simulink model "SimulArm_Interpolate_V2"  (R2025b)
settings: Solver=VariableStepAuto  StartTime=0.0  StopTime=45  FixedStep=.02  RelTol=1e-3  AbsTol=1e-3  EnableMultiTasking=on
values from neighbouring files (symbols this model uses):
  C = U * V'    [DataCondition.m]
  g = 9.80665    [DataCondition.m]
  N = numel(raw)    [DataCondition.m]
  pitch_offset = 0    [DataCondition.m]
  rot_x_bicep = [rot_x_bicep_ramp; rot_x_bicep]    [DataCondition.m]
  rot_y_bicep = [zeros(n_ramp,1); rot_y_bicep]    [DataCondition.m]
  rot_y_wrist = [zeros(n_ramp,1); rot_y_wrist]    [DataCondition.m]
  rot_z_bicep = [zeros(n_ramp,1); rot_z_bicep]    [DataCondition.m]
  rot_z_wrist = [zeros(n_ramp,1); rot_z_wrist]    [DataCondition.m]
  shoulder_limit = 30    [DataCondition.m]
  time = [time_ramp; time_motion]    [DataCondition.m]
  yaw_offset = 0    [DataCondition.m]
undefined symbols (not defined in the file or in its folder): X, Y, Z
libraries: sm_lib x45, nesl_utility x24, aerolibconvert2 x10, simulink x1
(part 3 of 3)

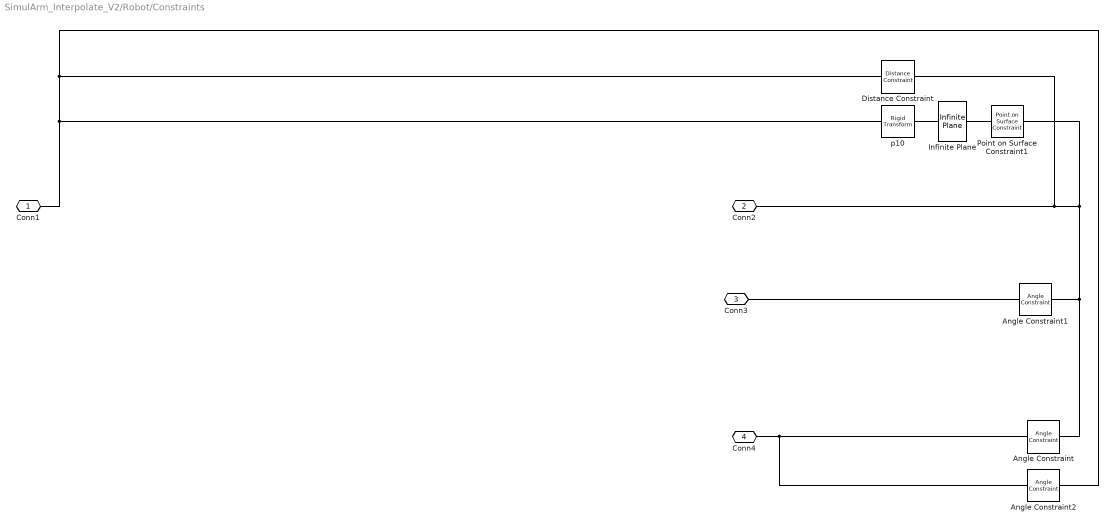
== system SimulArm_Interpolate_V2/Robot/Constraints ==
  Angle Constraint : sm_lib/Constraints/Angle Constraint  ConstraintType=Parallel  Angle=45  AngleUnits=deg  WrenchDir=FollowerOnBase  WrenchFrame=BaseFrame  SenseTorque=off  SenseSignedTorqueMagnitude=off
  Angle Constraint1 : sm_lib/Constraints/Angle Constraint  ConstraintType=Parallel  Angle=45  AngleUnits=deg  WrenchDir=FollowerOnBase  WrenchFrame=BaseFrame  SenseTorque=off  SenseSignedTorqueMagnitude=off
  Angle Constraint2 : sm_lib/Constraints/Angle Constraint  ConstraintType=Parallel  Angle=45  AngleUnits=deg  WrenchDir=FollowerOnBase  WrenchFrame=BaseFrame  SenseTorque=off  SenseSignedTorqueMagnitude=off
  Distance Constraint : sm_lib/Constraints/Distance Constraint  Distance=132  DistanceUnits=mm  WrenchDir=FollowerOnBase  WrenchFrame=BaseFrame  SenseForce=off  SenseSignedForceMagnitude=off
  Infinite Plane : sm_lib/Curves and Surfaces/Infinite Plane  GraphicType=Rectangle  GraphicPlaneWidth=1  GraphicPlaneWidthUnits=m  GraphicPlaneHeight=1  GraphicPlaneHeightUnits=m  GraphicVisPropType=SimpleVisualProperties  GraphicDiffuseColor=[0.5 0.5 0.5]  GraphicOpacity=.3  GraphicSpecularColor=[0.5 0.5 0.5 1.0]  GraphicAmbientColor=[0.15 0.15 0.15 1.0]  GraphicEmissiveColor=[0.0 0.0 0.0 1.0]  GraphicShininess=75
  Point on Surface Constraint1 : sm_lib/Constraints/Point on Surface Constraint  WrenchDir=FollowerOnBase  WrenchFrame=BaseFrame  SenseForce=off  SenseTorque=off
  p10 : sm_lib/Frames and Transforms/Rigid Transform  RotationMethod=None  FollAlignAxisA=+X  BaseAlignAxisA=+Y  FollAlignAxisB=+Y  BaseAlignAxisB=+Z  RotationStandardAxis=+Z  RotationAngle=0.0  RotationAngleUnits=deg  RotationArbitraryAxis=[0 0 1]  RotationSequenceAxes=FollowerAxes  RotationSequence=XZY  RotationSequenceAngles=-[90 -45 0]  RotationSequenceAnglesUnits=deg  RotationMatrix=[1 0 0; 0 1 0; 0 0 1]  Quaternion=[1 0 0 0]  TranslationMethod=Cartesian  TranslationCartesianOffset=[0 0 -132]  TranslationCartesianOffsetUnits=mm  TranslationStandardAxis=+Z  TranslationStandardOffset=0  TranslationStandardOffsetUnits=m  TranslationROffset=0  TranslationROffsetUnits=m  TranslationThetaOffset=0  TranslationThetaOffsetUnits=deg  TranslationZOffset=0  TranslationZOffsetUnits=m
  Conn1 : PMIOPort  Side=Left
  Conn2 : PMIOPort  Port=2  Side=Left
  Conn3 : PMIOPort  Port=3  Side=Left
  Conn4 : PMIOPort  Port=4  Side=Left
  connections:
  p10/LConn1 -- Conn1/RConn1 -- Angle Constraint2/RConn1 -- Distance Constraint/LConn1
  Infinite Plane/LConn1 -- p10/RConn1
  Point on Surface Constraint1/RConn1 -- Angle Constraint/RConn1 -- Angle Constraint1/RConn1 -- Conn2/RConn1 -- Distance Constraint/RConn1
  Infinite Plane/RConn1 -- Point on Surface Constraint1/LConn1
  Angle Constraint/LConn1 -- Conn4/RConn1 -- Angle Constraint2/LConn1
  Angle Constraint1/LConn1 -- Conn3/RConn1
